simulink model "fotflib"  (R2019b)
settings: Solver=ode45  StartTime=0.0  StopTime=10.0  RelTol=1e-3  EnableMultiTasking=on
model workspace (MAT data in the model file):
  a = -1.00008076451
undefined symbols (not defined in the file): G
libraries: cstblocks x6
settings Model: Creator=Professor Dingyu Xue  LastModifiedBy=xuedi
settings DataIOCC: LimitDataPoints=on  SaveFormat=Array  SignalLoggingSaveFormat=ModelDataLogs  ReturnWorkspaceOutputs=off
settings OptimizationCC: ExpressionDepthLimit=2147483647  LifeSpan=inf
settings DebuggingCC: UnderspecifiedInitializationDetection=Classic  MergeDetectMultiDrivingBlocksExec=none  SolverPrmCheckMsg=warning  FcnCallInpInsideContextMsg=warning  StateNameClashWarn=warning  SFUnexpectedBacktrackingDiag=warning  SFNoUnconditionalDefaultTransitionDiag=warning  SFExecutionAtInitializationDiag=none  ArithmeticOperatorsInVariantConditions=warning
settings HardwareCC: ProdBitPerPointer=32  ProdBitPerSizeT=32  ProdBitPerPtrDiffT=32  ProdLargestAtomicFloat=None  ProdIntDivRoundTo=Undefined  ProdEndianess=Unspecified  ProdWordSize=32  ProdHWDeviceType=32-bit Generic
settings ModelReferenceCC: PropagateSignalLabelsOutOfModel=off
settings SFSimCC: SimUseLocalCustomCode=off  CustomCodeUndefinedFunction=UseInterfaceOnly
settings RTWCC: RTWUseLocalCustomCode=off
settings CodeAppCC: StateflowObjectComments=on
settings GRTTargetCC: TargetLangStandard=C89/C90 (ANSI)  CombineOutputUpdateFcns=off  GRTInterface=on
settings ConfigComp: CovMetricSettings=dw  CovSaveCumulativeToWorkspaceVar=on  CovSaveSingleToWorkspaceVar=on  CovExternalEMLEnable=off

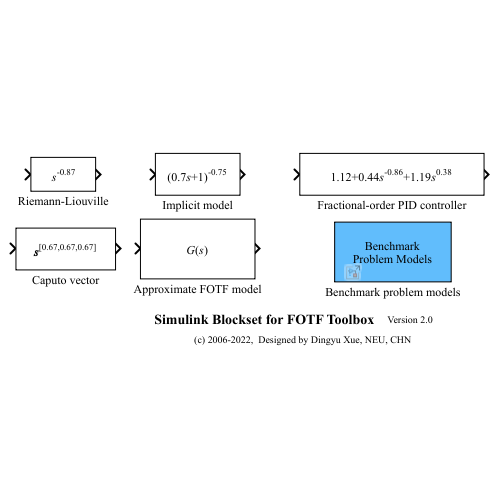
[thumbnail: Simulink's stored preview of the top-level diagram]
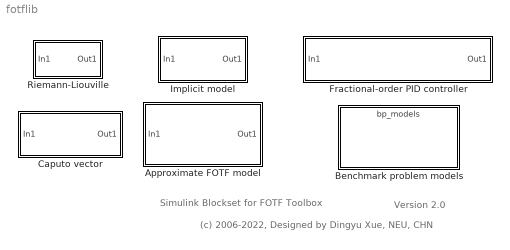
== system fotflib ==
  note: Version 2.0
  note: Simulink Blockset for FOTF Toolbox
  note: (c) 2006-2022, Designed by Dingyu Xue, NEU, CHN
  Approximate FOTF model : Subsystem  mask{na=[2.2 0.9 0], a=[0.8 0.5 1], nb=0, b=1, ww=[1e-4 1e4], N=11, kFilter=Oustaloup filter, T=0}
      mask prompts: na "Orders of the denominator"; a "Coefficients of the denominator"; nb "Orders of the numerator"; b "Coefficients of the numerator"; ww "Interested frequency range [wb wh]"; N "Filter order"; kFilter "Types of the filter"; T "Delay constant T"
      mask init:
      | if isa(na,'fotf'), G=na; 
      |    else
      |       if length(na)~=length(a)
      |          errordlg('Error','Mismatch on the denominator'), 
      |       end
      |       if length(b)~=length(nb)
      |          errordlg('Error','Mismatch on the numerator'), 
      |       end
      |       G=fotf(a,na,b,nb);
      |   end
      |   switch kFilter, case 1, str='ousta_fod'; 
      |      case 2, str='new_fod'; case 3, str='matsude_fod';
      |   end
      |   wb=ww(1); wh=ww(2); G1=high_order(G,str,wb,wh,N); [n,m]=size(G1);
      |   G1.ioDelay=T;
      mask TypeOptions kFilter: Oustaloup filter | Modified Oustaloup filter
      mask Display:
      | %disp('Fractional-order\ntransfer function')
      | if n*m>1
      |    disp('{\bm\itG}({\its})','texmode','on')
      | else
      |    disp('{\itG}({\its})','texmode','on')
      | end
  Benchmark problem models : ModelReference  ModelNameDialog=bp_models  SimulationMode=Normal  ModelReferenceVersion=2.0
      mask Display: disp('Benchmark\nProblem Models')
  Caputo vector : Subsystem  mask{gam=0.67, ww=[1e-4 1e4], N=11, M=3, x0=[3;2;1]}
      mask prompts: gam "Derivative order gamma"; ww "Frequency range [wb,wh]"; N "Approximation order N"; M "Dimension M"; x0 "Initial condition x0"
      mask init:
      | wb=ww(1); wh=ww(2); stri=[];
      | if length(gam)==1, gam=gam*ones(M,1); end
      | for i=1:M
      |     G(i,1)=ousta_fod(1-gam(i),N,wb,wh); stri=[stri,num2str(gam(i)),','];
      | end
      | str=['{\bf{\its}}^{[' stri(1:end-1) ']}'];
      | svec2sl(gam);
      mask Display: disp(str,'texmode','on')
  Fractional-order PID controller : Subsystem  mask{Kp=1.1202, II=[0.4391 0.8647], DD=[1.1907 0.3844], N=11, ww=[1e-4 1e4], kFilter=Oustaloup filter}
      mask prompts: Kp "Proportional Kp"; II "Integral [Ki lam]"; DD "Differentiation [Kd mu]"; N "Filter order"; ww "Interested frequency range [wb wh]"; kFilter "Types of the filter"
      mask init:
      | if isa(Kp,'fotf'), a=Kp;
      |    lam=a.den.na; mu=a.num.na; mu=mu(1)-lam; b=a.num.a; Kd=b(1); Kp=b(2); Ki=b(3);
      | else, II=[II 1]; DD=[DD 1]; Ki=II(1); lam=II(2); Kd=DD(1); mu=DD(2); end
      | s=fotf('s'); a=Kp+Ki/s^lam+Kd*s^mu/(0.001*s+1);
      | Gc=high_order(a,'ousta_fod',ww(1),ww(2),N);
      | if abs(Ki)>0, sI=[sprintf('%.2f',Ki),'{\its}^{' sprintf('%.2f',-lam), '}']; end
      | if abs(Kd)>0, sD=[sprintf('%.2f',Kd),'{\its}^{' sprintf('%.2f',mu), '}']; end
      | str=sprintf('%.2f',Kp);
      | if abs(Ki)>0, if sI(1)~='-', sI=['+' sI]; end, str=[str,sI]; end
      | if abs(Kd)>0, if sD(1)~='-', sD=['+' sD]; end, str=[str,sD]; end
      mask TypeOptions kFilter: Oustaloup filter | Modified Oustaloup filter
      mask Display: disp(str,'texmode','on')
  Implicit model : Subsystem  mask{tau=0.7, nu=0.75, ww=[1e-3 1e3], N=7}
      mask prompts: tau "Time constant tau"; nu "power nu"; ww "Frequency range ww"; N "Filter order"
      mask Display:
      | str=['(' num2str(tau) '{\its}+1)^{' num2str(-nu) '}'];
      | disp(str,'texmode','on')
  "Riemann-Liouville " : Subsystem  mask{gam=-0.87, ww=[1e-3, 1e3], n=5, kF1=off, kF=Oustaloup filter}
      mask prompts: gam "Derivative order gamma"; ww "Frequency range [wb,wh]"; n "Apprixmation order"; kF1 "Is a low-pass filter required?"; kF "Filter type"
      mask init:
      | wb=ww(1); wh=ww(2); 
      | if isnumeric(gam), str=['{\its}^{' num2str(gam) '}']; 
      | else, str='{\its}^{\gamma}'; end
      | if kF==1, G=ousta_fod(gam,n,wb,wh);
      | elseif kF==2, G=new_fod(gam,n,wb,wh); 
      | else, G=matsuda_fod(gam,n,wb,wh); end
      | T=1/wh; if kF1==1, G=G*tf(1,[T 1]); end
      mask TypeOptions kF: Oustaloup filter | Modified Oustaloup filter | Matsuda-Fujii filter
      mask Display: disp(str,'texmode','on')

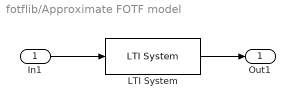
== system fotflib/Approximate FOTF model ==
  In1 : Inport
  LTI System : cstblocks/LTI System  sys=G1  IC=[]
  Out1 : Outport
  wires:
  In1/1 -> LTI System/1
  LTI System/1 -> Out1/1

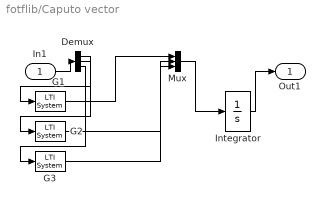
== system fotflib/Caputo vector ==
  In1 : Inport
  Demux : Demux  Outputs=3
  G1 : cstblocks/LTI System  sys=G(1)  IC=[]
  G2 : cstblocks/LTI System  sys=G(2)  IC=[]
  G3 : cstblocks/LTI System  sys=G(3)  IC=[]
  Integrator : Integrator  InitialCondition=x0
  Mux : Mux  Inputs=3
  Out1 : Outport
  wires:
  Demux/1 -> G1/1
  G1/1 -> Mux/1
  Demux/2 -> G2/1
  G2/1 -> Mux/2
  Demux/3 -> G3/1
  G3/1 -> Mux/3
  Integrator/1 -> Out1/1
  Mux/1 -> Integrator/1
  In1/1 -> Demux/1

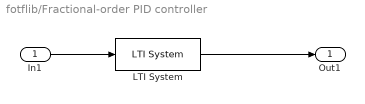
== system fotflib/Fractional-order PID controller ==
  In1 : Inport
  LTI System : cstblocks/LTI System  sys=Gc  IC=[]
  Out1 : Outport
  wires:
  LTI System/1 -> Out1/1
  In1/1 -> LTI System/1

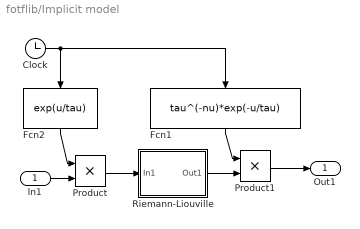
== system fotflib/Implicit model ==
  In1 : Inport
  Clock : Clock
  Fcn1 : Fcn  Expr=tau^(-nu)*exp(-u/tau)
  Fcn2 : Fcn  Expr=exp(u/tau)
  Product : Product
  Product1 : Product
  "Riemann-Liouville " : Subsystem  mask{gam=-nu, ww=ww, n=N, kF1=on, kF=Oustaloup filter}
      mask prompts: gam "Derivative order gamma"; ww "Frequency range [wb,wh]"; n "Apprixmation order"; kF1 "Is a low-pass filter required?"; kF "Filter type"
      mask init:
      | wb=ww(1); wh=ww(2); 
      | if kF==1, G=ousta_fod(gam,n,wb,wh);
      | else, G=new_fod(gam,n,wb,wh); end
      | G=tf(G); num=G.num{1}; den=G.den{1}; T=1/wh; 
      | if isnumeric(gam), str=['{\its}^{' num2str(gam) '}']; 
      | else, str='{\its}^{gam}'; end
      | if kF1==1, G=G*tf(1,[T 1]); end
      mask TypeOptions kF: Oustaloup filter | Modified Oustaloup filter | Matsuda-Fujii filter
      mask Display: disp(str,'texmode','on')
  Out1 : Outport
  wires:
  Clock/1 -> Fcn1/1, Fcn2/1
  Fcn1/1 -> Product1/1
  "Riemann-Liouville "/1(Out1) -> Product1/2
  Product/1 -> "Riemann-Liouville "/1(In1)
  Fcn2/1 -> Product/1
  In1/1 -> Product/2
  Product1/1 -> Out1/1

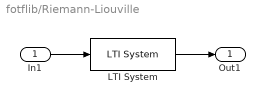
== system fotflib/Riemann-Liouville  ==
  In1 : Inport
  LTI System : cstblocks/LTI System  sys=G  IC=[]
  Out1 : Outport
  wires:
  LTI System/1 -> Out1/1
  In1/1 -> LTI System/1

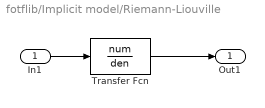
== system fotflib/Implicit model/Riemann-Liouville  ==
  In1 : Inport
  Transfer Fcn : TransferFcn  Numerator=num  Denominator=den
  Out1 : Outport
  wires:
  In1/1 -> Transfer Fcn/1
  Transfer Fcn/1 -> Out1/1
